simulink model "PIlow1"  (R2025a)
settings: Solver=VariableStepAuto  StartTime=0.0  StopTime=0.02  MaxStep=1e-9  RelTol=1e-3
libraries: spsVoltageMeasurementLib x5, spsSeriesRLCBranchLib x4, spsCurrentMeasurementLib x4, spsDiodeLib x2, spsMosfetLib x2, spsDCVoltageSourceLib x1, spsLinearTransformerLib x1, sps_lib x1
settings Model: Creator=FCH  LastModifiedBy=FCH
settings DataIOCC: ReturnWorkspaceOutputs=off

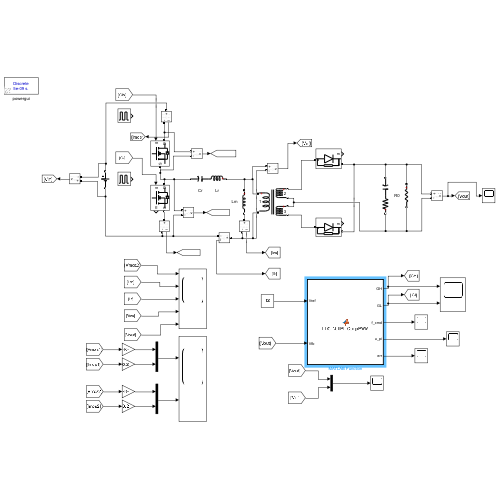
[thumbnail: Simulink's stored preview of the top-level diagram]
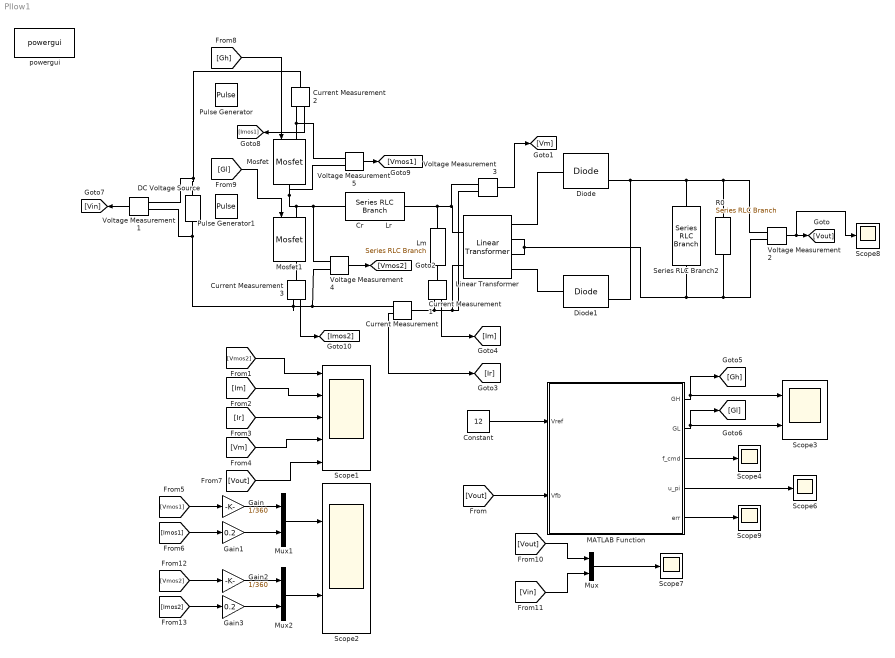
== system PIlow1 ==
  Constant : Constant  Value=12
  Cr           Lr : spsSeriesRLCBranchLib/Series RLC Branch  LConnTagsString=__new0  RConnTagsString=__new0  BranchType=LC  Resistance=1  Inductance=65.406e-6  SetiL0=off  InitialCurrent=0  Capacitance=38.728e-9  Setx0=off  InitialVoltage=0  Measurements=None
  Current Measurement{,1..3} (4 alike) : spsCurrentMeasurementLib/Current Measurement  PhasorSimulation=off  OutputType=Complex  PSBequivalent=0
  DC Voltage Source : spsDCVoltageSourceLib/DC Voltage Source  Amplitude=400  Measurements=None
  Diode : spsDiodeLib/Diode  Ron=0.001  Lon=0  Vf=0.8  IC=0  UseSnubber=0  Rs=500  Cs=250e-9  Measurements=on
  Diode1 : spsDiodeLib/Diode  Ron=0.001  Lon=0  Vf=0.8  IC=0  UseSnubber=0  Rs=500  Cs=250e-9  Measurements=on
  Gain : Gain  Gain=1/360
  Gain1 : Gain  Gain=0.2
  Gain2 : Gain  Gain=1/360
  Gain3 : Gain  Gain=0.2
  Linear Transformer : spsLinearTransformerLib/Linear Transformer  UNITS=SI  NominalPower=[ 250e2 180e6 ]  winding1=[16 0 0]  winding2=[1 0 0]  ThreeWindings=on  winding3=[1 0 0]  RmLm=[Inf Inf]  Measurements=None  DataType=on
  Lm : spsSeriesRLCBranchLib/Series RLC Branch  LConnTagsString=__new0  RConnTagsString=__new0  BranchType=L  Resistance=1  Inductance=392.437e-6  SetiL0=off  InitialCurrent=0  Capacitance=1e-6  Setx0=off  InitialVoltage=0  Measurements=None
  MATLAB Function : MATLAB Function  TreatAsAtomicUnit=on
  Mosfet : spsMosfetLib/Mosfet  Ron=0.1  Lon=0  Rd=0.01  Vfd=0  IC=0  Rs=200  Cs=4.7e-9  Measurements=off
  Mosfet1 : spsMosfetLib/Mosfet  Ron=0.1  Lon=0  Rd=0.01  Vfd=0  IC=0  Rs=200  Cs=4.7e-9  Measurements=on
  Mux : Mux  Inputs=2
  Mux1 : Mux  Inputs=2
  Mux2 : Mux  Inputs=2
  Pulse Generator : DiscretePulseGenerator  PulseType=Time based  Period=1/100e3  PulseWidth=50
  Pulse Generator1 : DiscretePulseGenerator  PulseType=Time based  Period=1/100e3  PulseWidth=50  PhaseDelay=180/360*1/100e3
  R0 : spsSeriesRLCBranchLib/Series RLC Branch  LConnTagsString=__new0  RConnTagsString=__new0  BranchType=R  Resistance=100  Inductance=1e-3  SetiL0=off  InitialCurrent=0  Capacitance=1e-6  Setx0=off  InitialVoltage=0  Measurements=Branch voltage
  Scope1 : Scope  NumInputPorts=5
      settings: ActiveDisplayYMinimum=-50.001884345924758  ActiveDisplayYMaximum=450.00165939733819
  Scope2 : Scope  NumInputPorts=2
      settings: ActiveDisplayYMinimum=-2.2545286858856493  ActiveDisplayYMaximum=1.9388480706148599
  Scope3 : Scope  NumInputPorts=2
      settings: ActiveDisplayYMinimum=-1  ActiveDisplayYMaximum=1  DataLoggingVariableName=ScopeData3
  Scope{4,6..9} (5 alike) : Scope
      Scope4 settings: ActiveDisplayYMinimum=247002.01307117686  ActiveDisplayYMaximum=247384.68643605898  DataLoggingVariableName=ScopeData4
      Scope6 settings: ActiveDisplayYMinimum=-2.969655937212309  ActiveDisplayYMaximum=0.86494119466968022  DataLoggingVariableName=ScopeData6
      Scope7 settings: ActiveDisplayYMinimum=-44.999999999999972  ActiveDisplayYMaximum=404.99999999999994  DataLoggingVariableName=ScopeData2
      Scope8 settings: ActiveDisplayYMinimum=11.887564091641098  ActiveDisplayYMaximum=12.102438131972715  DataLoggingVariableName=U_output
      Scope9 settings: ActiveDisplayYMinimum=-0.21612308169830813  ActiveDisplayYMaximum=-0.19327697437090471  DataLoggingVariableName=ScopeData8
  Series RLC Branch2 : spsSeriesRLCBranchLib/Series RLC Branch  LConnTagsString=__new0  RConnTagsString=__new0  BranchType=RC  Resistance=0.01  Inductance=1e-3  SetiL0=off  InitialCurrent=0  Capacitance=1e-5  Setx0=off  InitialVoltage=0  Measurements=None
  Voltage Measurement{1..5} (5 alike) : spsVoltageMeasurementLib/Voltage Measurement  PhasorSimulation=off  OutputType=Complex  PSBequivalent=0
  powergui : sps_lib/powergui  Priority=1  SimulationMode=Discrete  SampleTime=1/(200e6)  frequency=60  Iterations=50  frequencyindice=0  Pbase=100e6  ErrMax=1e-4  UnitsV=kV  UnitsW=MW  buscounter=0  FunctionMessages=off  echomessages=off  EnableUseOfTLC=off  CurrentSourceSwitches=off  DisableSnubberDevices=off  DisableRonSwitches=off  DisableVfSwitches=off  DisplayEquations=off  AutomaticDiscreteSolvers=off  SolverType=Tustin/Backward Euler (TBE)  Interpol=off  ExternalGateDelay=off  methode=off  Ts=100  x0status=blocks  SPID=on  SwTol=0  HookPort=off  NonlinearTolerance=1e-4  nMaxIteration=100  ContinueOnMaxIteration=off  RestoreLinks=warning  ResistiveCurrentMeasurement=off  Frange=[0:2:500]  Ylog=off  Xlog=on  ShowGrid=off  save=off  variable=ZData  structure=0  ZoomFFT=off  StartTime=0.0  cycles=1  DisplayStyle=1  fundamental=60  FreqAxis=off  MaxFrequency=1000  frequencyindicesteady=1  RmsSteady=1  display=off
  wires:
  Voltage Measurement2/1 -> Scope8/1, [Vout]
  Constant/1 -> MATLAB Function/1(Vref)
  [Vout] -> MATLAB Function/2(Vfb)
  MATLAB Function/1(GH) -> [Gh], Scope3/1
  MATLAB Function/2(GL) -> [Gl], Scope3/2
  MATLAB Function/4(u_pi) -> Scope6/1
  MATLAB Function/3(f_cmd) -> Scope4/1
  MATLAB Function/5(err) -> Scope9/1
  Voltage Measurement3/1 -> [Vm]
  Voltage Measurement4/1 -> [Vmos2]
  Current Measurement/1 -> [Ir]
  Current Measurement1/1 -> [Im]
  [Vmos2] -> Scope1/1
  [Im] -> Scope1/2
  [Ir] -> Scope1/3
  [Vm] -> Scope1/4
  [Vout] -> Scope1/5
  Mux/1 -> Scope7/1
  [Vout] -> Mux/1
  Voltage Measurement1/1 -> [Vin]
  [Vin] -> Mux/2
  Current Measurement2/1 -> [Imos1]
  Voltage Measurement5/1 -> [Vmos1]
  Current Measurement3/1 -> [Imos2]
  [Vmos1] -> Gain/1
  [Imos1] -> Gain1/1
  Mux1/1 -> Scope2/1
  [Vmos2] -> Gain2/1
  [Imos2] -> Gain3/1
  Mux2/1 -> Scope2/2
  Gain/1 -> Mux1/1
  Gain1/1 -> Mux1/2
  Gain2/1 -> Mux2/1
  Gain3/1 -> Mux2/2
  [Gh] -> Mosfet/1
  [Gl] -> Mosfet1/1
  connections:
  DC Voltage Source/RConn1 -- Voltage Measurement1/LConn2 -- Current Measurement2/LConn1
  Mosfet/RConn1 -- Voltage Measurement4/LConn1 -- Cr           Lr/RConn1 -- Mosfet1/LConn1 -- Voltage Measurement5/LConn2
  Lm/RConn1 -- Current Measurement1/LConn1
  Cr           Lr/LConn1 -- Voltage Measurement3/LConn1 -- Linear Transformer/LConn1 -- Lm/LConn1
  Linear Transformer/RConn1 -- Diode/LConn1
  Diode/RConn1 -- Diode1/RConn1 -- Series RLC Branch2/RConn1 -- R0/LConn1 -- Voltage Measurement2/LConn1
  R0/RConn1 -- Voltage Measurement2/LConn2 -- Linear Transformer/RConn2 -- Linear Transformer/RConn3 -- Series RLC Branch2/LConn1
  Linear Transformer/RConn4 -- Diode1/LConn1
  Current Measurement/RConn1 -- Voltage Measurement1/LConn1 -- DC Voltage Source/LConn1 -- Current Measurement3/RConn1 -- Voltage Measurement4/LConn2
  Linear Transformer/LConn2 -- Voltage Measurement3/LConn2 -- Current Measurement1/RConn1 -- Current Measurement/LConn1
  Current Measurement2/RConn1 -- Mosfet/LConn1 -- Voltage Measurement5/LConn1
  Mosfet1/RConn1 -- Current Measurement3/LConn1

== matlab function PIlow1/MATLAB Function ==
  data: Vref input; GH output; Vfb input; GL output; f_cmd output; u_pi output; err output
function [GH, GL, f_cmd, u_pi, err] = LLC_VoltPI_CompPWM(Vref, Vfb)
%#codegen
% LLC 变换器 PI 电压闭环 + 互补 PWM 驱动（变频控制）
% 去掉 PI 限幅，但保留最小频率保护

%% ========= 用户参数 =========

% 1) PWM/函数调用步长：必须与你的 MATLAB Function 实际离散步长一致
Ts_pwm = 1/(200e6);

% 2) 电压环更新周期
T_ctrl = 10/(200e6);

% 3) PI 参数
Kp = 30;
Ki = 0;

% 4) LLC 频率范围
f_min  = 30e3;
f_max  = 300e3;
f_init = 100e3;

% 5) 启动阶段固定频率时间
t_startup = 2e-3;

% 6) 死区时间
t_dead = 200e-9;

% 7) 反馈低通滤波时间常数
tau_vfb = 0.5e-3;

% 8) 频率命令每次控制更新的最大变化量
df_max = 50000000;

% 9) LLC 调频方向
freq_inverse = true;

%% ========= 持久变量 =========
persistent ui ...
           t_half leg dead_t ...
           ctrl_t run_t ...
           vfb_f ...
           f_cmd_hold ...
           u_pi_hold err_hold ...
           u_pi_init

if isempty(ui)
    % 根据初始频率反算初始控制量
    if freq_inverse
        u_norm_init = (f_max - f_init) / (f_max - f_min);
    else
        u_norm_init = (f_init - f_min) / (f_max - f_min);
    end

    u_pi_init = 2.0 * u_norm_init - 1.0;
    ui = u_pi_init;

    t_half     = 0.0;
    leg        = int8(0);
    dead_t     = 0.0;

    ctrl_t     = 0.0;
    run_t      = 0.0;

    vfb_f      = Vfb;
    f_cmd_hold = f_init;

    u_pi_hold  = u_pi_init;
    err_hold   = Vref - Vfb;
end

%% ========= 默认输出保持 =========
f_cmd = f_cmd_hold;
u_pi  = u_pi_hold;
err   = err_hold;

%% ========= 运行时间 =========
run_t = run_t + Ts_pwm;

%% ========= 慢速电压环 =========
ctrl_t = ctrl_t + Ts_pwm;

if ctrl_t >= T_ctrl
    ctrl_t = ctrl_t - T_ctrl;

    % ---- 1) 反馈低通滤波 ----
    alpha = T_ctrl / (tau_vfb + T_ctrl);
    vfb_f = vfb_f + alpha * (Vfb - vfb_f);

    % 使用滤波后反馈计算误差
    err = Vref - vfb_f;
    err_hold = err;

    % ---- 2) 启动阶段：固定初始频率 ----
    if run_t < t_startup
        u_pi = u_pi_init;
        u_pi_hold = u_pi;
        f_cmd_hold = f_init;

    else
        % ---- 3) PI 计算：去掉 PI 限幅和抗饱和 ----
        up = Kp * err;
        ui = ui + Ki * T_ctrl * err;
        u_pi = up + ui;
        u_pi_hold = u_pi;

        % ---- 4) PI 输出映射到频率 ----
        u_norm = 0.5 + 0.5 * u_pi;

        if freq_inverse
            f_target = f_max - u_norm * (f_max - f_min);
        else
            f_target = f_min + u_norm * (f_max - f_min);
        end

        % ---- 5) 频率限速 ----
        df = f_target - f_cmd_hold;

        if df > df_max
            df = df_max;
        elseif df < -df_max
            df = -df_max;
        end

        f_cmd_hold = f_cmd_hold + df;

        % ---- 6) 只保留最小频率保护 ----
        if f_cmd_hold < f_min
            f_cmd_hold = f_min;
        end
    end

    f_cmd = f_cmd_hold;
end

%% ========= 根据频率命令生成 50% 占空互补驱动 =========
T_half = 1.0 / (2.0 * f_cmd_hold);

t_half = t_half + Ts_pwm;

while t_half >= T_half
    t_half = t_half - T_half;
    leg    = bitxor(leg, int8(1));
    dead_t = t_dead;
end

%% ========= 死区 + 互补输出 =========
if dead_t > 0
    dead_t = dead_t - Ts_pwm;
    GH = false;
    GL = false;
else
    if leg == 0
        GH = true;
        GL = false;
    else
        GH = false;
        GL = true;
    end
end

end
